simulink model "popul"  (Simulink 8.7)
settings: Solver=ode3  StartTime=0.0  StopTime=20  FixedStep=0.0001  RelTol=1e-3
settings Model: Creator=Dinis  LastModifiedBy=Dinis
settings DataIOCC: LimitDataPoints=off  SaveFormat=Dataset
settings DebuggingCC: UnderspecifiedInitializationDetection=Simplified  MergeDetectMultiDrivingBlocksExec=error
settings HardwareCC: ProdBitPerPointer=64  ProdLargestAtomicFloat=Float  ProdIntDivRoundTo=Zero  ProdEndianess=LittleEndian  ProdHWDeviceType=Specified
settings ModelReferenceCC: PropagateSignalLabelsOutOfModel=on
settings ConfigComp: CovModelRefEnable=off

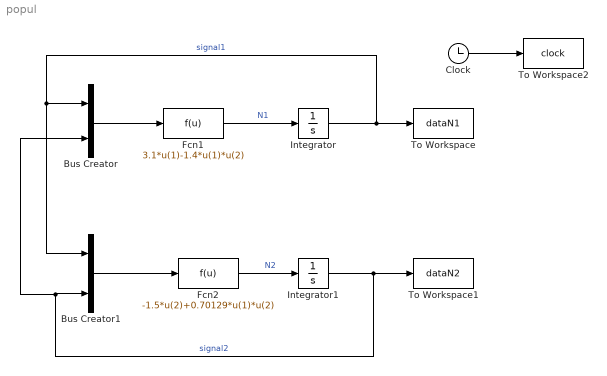
== system popul ==
  Bus Creator : BusCreator  Inputs=2
  Bus Creator1 : BusCreator  Inputs=2
  Clock : Clock
  Fcn1 : Fcn  Expr=3.1*u(1)-1.4*u(1)*u(2)
  Fcn2 : Fcn  Expr=-1.5*u(2)+0.70129*u(1)*u(2)
  Integrator : Integrator  InitialCondition=4
  Integrator1 : Integrator  InitialCondition=1.5982
  To Workspace : ToWorkspace  VariableName=dataN1  SampleTime=-1
  To Workspace1 : ToWorkspace  VariableName=dataN2  SampleTime=-1
  To Workspace2 : ToWorkspace  VariableName=clock  SampleTime=-1
  wires:
  Bus Creator1/1 -> Fcn2/1
  Fcn2/1 -> Integrator1/1  "N2"
  Fcn1/1 -> Integrator/1  "N1"
  Bus Creator/1 -> Fcn1/1
  Integrator/1 -> Bus Creator1/1, Bus Creator/1, To Workspace/1  "signal1"
  Integrator1/1 -> Bus Creator/2, Bus Creator1/2, To Workspace1/1  "signal2"
  Clock/1 -> To Workspace2/1
